simulink model "SixDOFSim"  (R2020b)
settings: Solver=VariableStepAuto  StartTime=0.0  StopTime=80  RelTol=1e-3
values from neighbouring files (symbols this model uses):
  A = sys_ol.A    [cost_condition_number.m]    (also in cost_coupling_control.m; cost_filter.m; coupling_control_scratch.m = sys.A; coupling_control_scratch2.m = sys.A)
  B = sys_ol.B    [cost_condition_number.m]    (also in cost_coupling_control.m; cost_filter.m; coupling_control_scratch.m = sys.B; coupling_control_scratch2.m = sys.B)
  C_tilde = zeros(size(C,1), size(A,1))    [SixDOFModel.m]    (also in cost_condition_number.m = struct_cond.C_tilde; cost_coupling_control.m = struct_cond.C_tilde; cost_filter.m = struct_cond.C_tilde; coupling_controller.m = T*C_resort)
  deltaX_init = Tx\deltaX_init    [SixDOFModel.m]    (also in coupling_controller_main.m = X_init-X_ap_simulink)
  eta_max = 15*pi/180    (= 0.261799387799)    [SixDOFModel.m]    (also in coupling_controller_main.m = 0.174532925199; load_messung_one_massmodel.m = 0.174532925199)
  eta_min = - 30*pi/180    (= -0.523598775598)    [SixDOFModel.m]    (also in coupling_controller_main.m = -0.436332312999; load_messung_one_massmodel.m = -0.436332312999)
  F = real(F)    [coupling_control_scratch.m]    (also in coupling_control_scratch2.m; coupling_controller.m = Kopt{end}; coupling_controller_main.m = -inv(C*(Ak\B)); coupling_controller_philipp.m = -inv(C*(Ak\B)))
  F_mod = F_ent(:,1:p/2)    [SixDOFModel.m]    (also in coupling_controller_main.m = F1*Q_mod; coupling_controller_philipp.m = F1*Q_mod; script_kein_theta_verk.m = F1*Q_mod)
  K_coupling = inv(Dstar)*compR    [SixDOFModel.m]    (also in coupling_controller_main.m = Kopt{1}; coupling_controller_philipp.m = Kopt{1}; script_kein_theta_verk.m = Kopt{1})
  latlon_init = [0;0]    [SixDOFModel.m]    (also in create_multi_model.m)
  m = i-1    [coupling_control_scratch.m]    (also in coupling_control_scratch2.m; defineABC.m = size(B_1,2) + size(B_2,2); implicit_linmod.m = length(U_ap); initializeParameters.m = 120000)
  noise_weight = [10 10 10 1 1 1 1 1 10 10 10 10 1 1 1 1 1 10]'    [SixDOFModel.m]
  P_e_init_1 = [0;0;-h_init_1]    [SixDOFModel.m]    (also in create_multi_model.m)
  P_e_init_2 = [0;0;-h_init_2]    [SixDOFModel.m]    (also in create_multi_model.m)
  q = X(5)    [nonlinear_6DOF.m]    (also in normieren.m = size (C,1))
  r = 5    [coupling_controller.m]    (also in coupling_controller_main.m = 100; coupling_controller_philipp.m = 200; nonlinear_6DOF.m = X(6); polgebiet.m = a2)
  sigmaf_max = 20*pi/180    (= 0.349065850399)    [SixDOFModel.m]    (also in coupling_controller_main.m; load_messung_one_massmodel.m)
  sigmaf_min = 0.5*pi/180    (= 0.00872664625997)    [SixDOFModel.m]    (also in coupling_controller_main.m; load_messung_one_massmodel.m)
  Tu = eye(size(B,2))    [SixDOFModel.m]    (also in normieren.m = zeros(p,p))
  Tx = eye(n)    [SixDOFModel.m]    (also in normieren.m = diag([200 15 50 0.1 0.1 0.1 45*pi/180 45*pi/180 10000 200 15)
  Ty = eye(size(C,1))    [SixDOFModel.m]    (also in normieren.m = zeros(q,q))
  U_ap = Tu\U_ap    [SixDOFModel.m]    (also in coupling_controller_main.m = AP(1,1).U_ap; create_multi_model.m = [U_ap_1;U_ap_2]; fsolve_trim.m = ap(11:14); trimValues.m = Z_ap(11:14))
  W_ap = W_ap(1:4)    [SixDOFModel.m]    (also in coupling_controller_philipp.m = (C*X_ap_simulink)')
  X_ap = [X_ap_1;X_ap_2]    [SixDOFModel.m]    (also in coupling_controller_main.m = AP(1,1).X_ap; create_multi_model.m; fsolve_trim.m = ap(1:10); trimValues.m = Z_ap(1:10))
  X_ap_simulink = Tx\X_ap_simulink    [SixDOFModel.m]    (also in coupling_controller_main.m = AP(1,1).X_ap_simulink; create_multi_model.m = [X_ap(1:8);X_ap(10);X_ap(11:18);X_ap(20)])
  X_init = Tx\X_init    [SixDOFModel.m]    (also in cost_coupling_control.m = struct_cond.X_init; cost_filter.m = struct_cond.X_init; coupling_controller_main.m = X_ap_simulink; create_multi_model.m = [X_init_1; X_init_2])
  xi_max = 25*pi/180    (= 0.436332312999)    [SixDOFModel.m]    (also in coupling_controller_main.m; load_messung_one_massmodel.m)
  xi_min = - xi_max    (= -0.436332312999)    [SixDOFModel.m]    (also in coupling_controller_main.m; load_messung_one_massmodel.m)
  zita_max = 30*pi/180    (= 0.523598775598)    [SixDOFModel.m]    (also in coupling_controller_main.m; load_messung_one_massmodel.m)
  zita_min = - zita_max    (= -0.523598775598)    [SixDOFModel.m]    (also in coupling_controller_main.m; load_messung_one_massmodel.m)
undefined symbols (not defined in the file or in its folder): Earth, globalParameters, Light, MIL, WGS84
libraries: aerolibfltsims x24, aerolibtransform2 x4, aerolibwind2 x4, simulink x3, shared6dof x1, aerolibanim x1
(part 2 of 3)

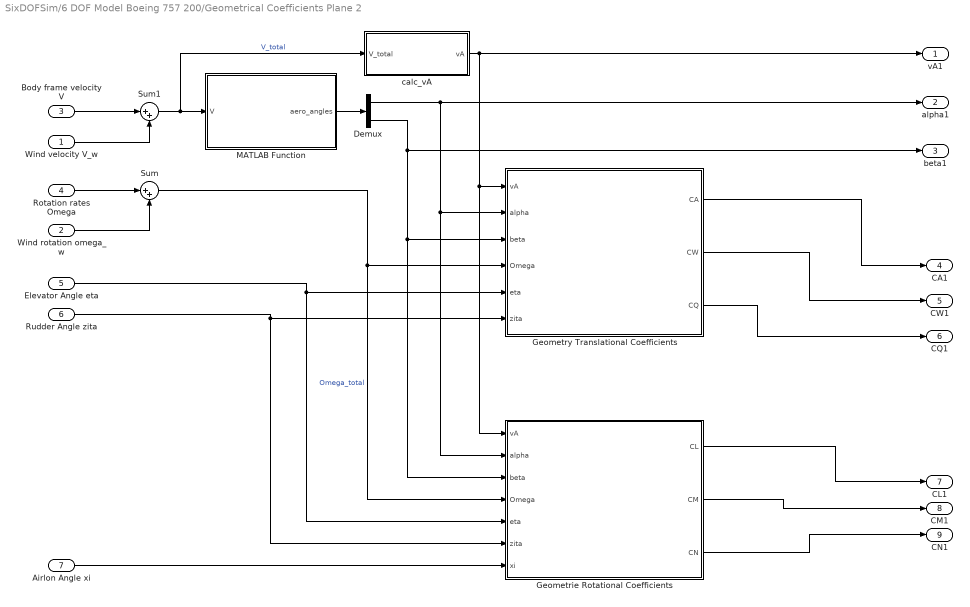
== system SixDOFSim/6 DOF Model Boeing 757 200/Geometrical Coefficients Plane 2 ==
  Wind velocity V_w : Inport
  Wind rotation omega_w : Inport  Port=2
  Body frame velocity V : Inport  Port=3
  Rotation rates Omega : Inport  Port=4
  Elevator Angle eta : Inport  Port=5
  Rudder Angle zita : Inport  Port=6
  Airlon Angle xi : Inport  Port=7
  Demux : Demux  Outputs=2
  Geometrie Rotational Coefficients : MATLAB Function  TreatAsAtomicUnit=on
  Geometry Translational Coefficients : MATLAB Function  TreatAsAtomicUnit=on
  MATLAB Function : MATLAB Function  TreatAsAtomicUnit=on
  Sum : Sum  Inputs=|++
  Sum1 : Sum  Inputs=|++
  calc_vA : MATLAB Function  TreatAsAtomicUnit=on
  vA1 : Outport
  alpha1 : Outport  Port=2
  beta1 : Outport  Port=3
  CA1 : Outport  Port=4
  CW1 : Outport  Port=5
  CQ1 : Outport  Port=6
  CL1 : Outport  Port=7
  CM1 : Outport  Port=8
  CN1 : Outport  Port=9
  wires:
  Airlon Angle xi/1 -> Geometrie Rotational Coefficients/7(xi)
  Geometrie Rotational Coefficients/2(CM) -> CM1/1
  Geometry Translational Coefficients/2(CW) -> CW1/1
  Rudder Angle zita/1 -> Geometrie Rotational Coefficients/6(zita), Geometry Translational Coefficients/6(zita)
  Geometry Translational Coefficients/1(CA) -> CA1/1
  Geometrie Rotational Coefficients/3(CN) -> CN1/1
  Geometry Translational Coefficients/3(CQ) -> CQ1/1
  Geometrie Rotational Coefficients/1(CL) -> CL1/1
  Elevator Angle eta/1 -> Geometrie Rotational Coefficients/5(eta), Geometry Translational Coefficients/5(eta)
  Body frame velocity V/1 -> Sum1/1
  Rotation rates Omega/1 -> Sum/1
  Wind velocity V_w/1 -> Sum1/2
  Wind rotation omega_w/1 -> Sum/2
  Sum1/1 -> calc_vA/1(V_total), MATLAB Function/1(V)  "V_total"
  MATLAB Function/1(aero_angles) -> Demux/1
  Demux/1 -> Geometrie Rotational Coefficients/2(alpha), Geometry Translational Coefficients/2(alpha), alpha1/1
  Demux/2 -> beta1/1, Geometrie Rotational Coefficients/3(beta), Geometry Translational Coefficients/3(beta)
  Sum/1 -> Geometrie Rotational Coefficients/4(Omega), Geometry Translational Coefficients/4(Omega)  "Omega_total"
  calc_vA/1(vA) -> vA1/1, Geometrie Rotational Coefficients/1(vA), Geometry Translational Coefficients/1(vA)

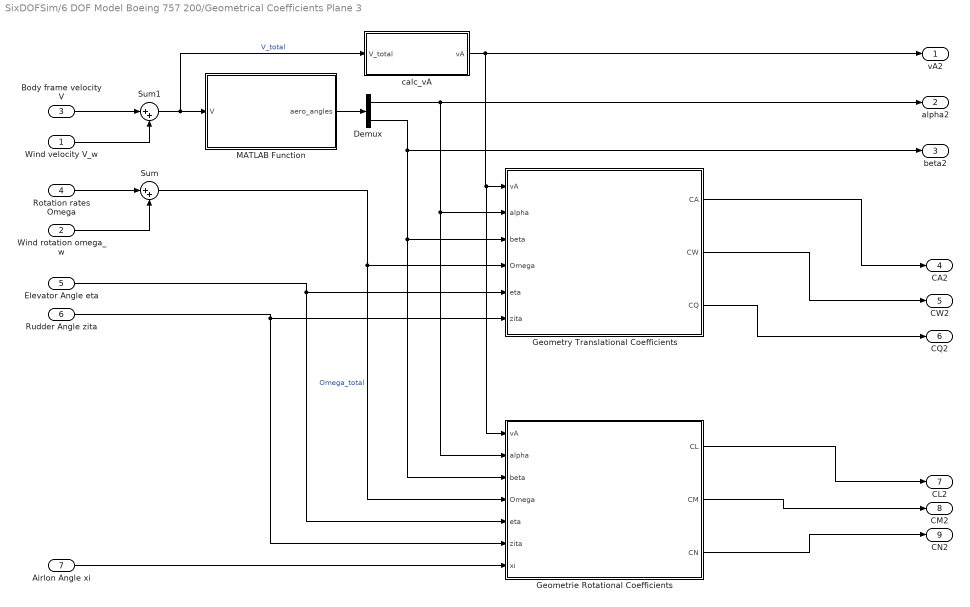
== system SixDOFSim/6 DOF Model Boeing 757 200/Geometrical Coefficients Plane 3 ==
  Wind velocity V_w : Inport
  Wind rotation omega_w : Inport  Port=2
  Body frame velocity V : Inport  Port=3
  Rotation rates Omega : Inport  Port=4
  Elevator Angle eta : Inport  Port=5
  Rudder Angle zita : Inport  Port=6
  Airlon Angle xi : Inport  Port=7
  Demux : Demux  Outputs=2
  Geometrie Rotational Coefficients : MATLAB Function  TreatAsAtomicUnit=on
  Geometry Translational Coefficients : MATLAB Function  TreatAsAtomicUnit=on
  MATLAB Function : MATLAB Function  TreatAsAtomicUnit=on
  Sum : Sum  Inputs=|++
  Sum1 : Sum  Inputs=|++
  calc_vA : MATLAB Function  TreatAsAtomicUnit=on
  vA2 : Outport
  alpha2 : Outport  Port=2
  beta2 : Outport  Port=3
  CA2 : Outport  Port=4
  CW2 : Outport  Port=5
  CQ2 : Outport  Port=6
  CL2 : Outport  Port=7
  CM2 : Outport  Port=8
  CN2 : Outport  Port=9
  wires:
  calc_vA/1(vA) -> Geometrie Rotational Coefficients/1(vA), Geometry Translational Coefficients/1(vA), vA2/1
  Sum/1 -> Geometry Translational Coefficients/4(Omega), Geometrie Rotational Coefficients/4(Omega)  "Omega_total"
  Demux/2 -> Geometry Translational Coefficients/3(beta), Geometrie Rotational Coefficients/3(beta), beta2/1
  Demux/1 -> alpha2/1, Geometry Translational Coefficients/2(alpha), Geometrie Rotational Coefficients/2(alpha)
  MATLAB Function/1(aero_angles) -> Demux/1
  Sum1/1 -> MATLAB Function/1(V), calc_vA/1(V_total)  "V_total"
  Wind rotation omega_w/1 -> Sum/2
  Wind velocity V_w/1 -> Sum1/2
  Rotation rates Omega/1 -> Sum/1
  Body frame velocity V/1 -> Sum1/1
  Elevator Angle eta/1 -> Geometry Translational Coefficients/5(eta), Geometrie Rotational Coefficients/5(eta)
  Geometrie Rotational Coefficients/1(CL) -> CL2/1
  Geometry Translational Coefficients/3(CQ) -> CQ2/1
  Geometrie Rotational Coefficients/3(CN) -> CN2/1
  Geometry Translational Coefficients/1(CA) -> CA2/1
  Rudder Angle zita/1 -> Geometry Translational Coefficients/6(zita), Geometrie Rotational Coefficients/6(zita)
  Geometry Translational Coefficients/2(CW) -> CW2/1
  Geometrie Rotational Coefficients/2(CM) -> CM2/1
  Airlon Angle xi/1 -> Geometrie Rotational Coefficients/7(xi)

== system SixDOFSim/6 DOF Model Boeing 757 200/Motion model Plain3 ==
  Omega : Inport
  V : Inport  Port=2
  Forces : Inport  Port=3
  Torque : Inport  Port=4
  Euler angles : Inport  Port=5
  Dynamics : Subsystem
  dV2 : Outport
  dOmega2 : Outport  Port=2
  dPhi2 : Outport  Port=3
  dxyh2 : Outport  Port=4
  vk2 : Outport  Port=5
  chsi2 : Outport  Port=6
  gamma2 : Outport  Port=7
  wires:
  Dynamics/7(gamma) -> gamma2/1
  Dynamics/6(chsi) -> chsi2/1
  Dynamics/5(vk) -> vk2/1
  Dynamics/4(dxyh) -> dxyh2/1
  Dynamics/3(dPhi) -> dPhi2/1
  Dynamics/1(dV) -> dV2/1
  V/1 -> Dynamics/2(V)
  Omega/1 -> Dynamics/1(Omega)
  Euler angles/1 -> Dynamics/5(Euler Angles( Phi))
  Torque/1 -> Dynamics/4(Torque)
  Forces/1 -> Dynamics/3(Forces)
  Dynamics/2(dOmega) -> dOmega2/1

== system SixDOFSim/6 DOF Model Boeing 757 200/Motion model Plane 2 ==
  Omega : Inport
  V : Inport  Port=2
  Forces : Inport  Port=3
  Torque : Inport  Port=4
  Euler angles : Inport  Port=5
  Dynamics : Subsystem
  dV1 : Outport
  dOmega1 : Outport  Port=2
  dPhi1 : Outport  Port=3
  dxyh1 : Outport  Port=4
  vk1 : Outport  Port=5
  chsi1 : Outport  Port=6
  gamma1 : Outport  Port=7
  wires:
  Dynamics/2(dOmega) -> dOmega1/1
  Forces/1 -> Dynamics/3(Forces)
  Torque/1 -> Dynamics/4(Torque)
  Euler angles/1 -> Dynamics/5(Euler Angles( Phi))
  Omega/1 -> Dynamics/1(Omega)
  V/1 -> Dynamics/2(V)
  Dynamics/1(dV) -> dV1/1
  Dynamics/3(dPhi) -> dPhi1/1
  Dynamics/4(dxyh) -> dxyh1/1
  Dynamics/5(vk) -> vk1/1
  Dynamics/6(chsi) -> chsi1/1
  Dynamics/7(gamma) -> gamma1/1

== system SixDOFSim/6 DOF Model Boeing 757 200/Rho ==
  h1 : Inport
  calc_rho : MATLAB Function  TreatAsAtomicUnit=on
  rho1 : Outport
  wires:
  h1/1 -> calc_rho/1(h)
  calc_rho/1(rho) -> rho1/1

== system SixDOFSim/6 DOF Model Boeing 757 200/Rho1 ==
  h2 : Inport
  calc_rho : MATLAB Function  TreatAsAtomicUnit=on
  rho2 : Outport
  wires:
  calc_rho/1(rho) -> rho2/1
  h2/1 -> calc_rho/1(h)

== system SixDOFSim/6 DOF Model Boeing 757 200/Stellgrößenbeschränkung ==
  eta_soll_1 : Inport
  sigmaf_soll_1 : Inport  Port=2
  xi_soll_1 : Inport  Port=3
  zita_soll_1 : Inport  Port=4
  Saturation airlon p1 : Saturate  UpperLimit=xi_max  LowerLimit=xi_min
  Saturation elevator p1 : Saturate  UpperLimit=eta_max  LowerLimit=eta_min
  Saturation rudder p1 : Saturate  UpperLimit=zita_max  LowerLimit=zita_min
  Saturation throttle p1 : Saturate  UpperLimit=sigmaf_max  LowerLimit=sigmaf_min
  eta_ist_1 : Outport
  sigmaf_ist_1 : Outport  Port=2
  xi_ist_1 : Outport  Port=3
  zita_ist_1 : Outport  Port=4
  wires:
  xi_soll_1/1 -> Saturation airlon p1/1
  zita_soll_1/1 -> Saturation rudder p1/1
  Saturation airlon p1/1 -> xi_ist_1/1
  Saturation elevator p1/1 -> eta_ist_1/1
  eta_soll_1/1 -> Saturation elevator p1/1
  Saturation throttle p1/1 -> sigmaf_ist_1/1
  sigmaf_soll_1/1 -> Saturation throttle p1/1
  Saturation rudder p1/1 -> zita_ist_1/1

== system SixDOFSim/6 DOF Model Boeing 757 200/Stellgrößenbeschränkung 2 ==
  eta_soll_2 : Inport
  sigmaf_soll_2 : Inport  Port=2
  xi_soll_2 : Inport  Port=3
  zita_soll_2 : Inport  Port=4
  Saturation airlon p2 : Saturate  UpperLimit=xi_max  LowerLimit=xi_min
  Saturation elevator p2 : Saturate  UpperLimit=eta_max  LowerLimit=eta_min
  Saturation rudder p2 : Saturate  UpperLimit=zita_max  LowerLimit=zita_min
  Saturation throttle p2 : Saturate  UpperLimit=sigmaf_max  LowerLimit=sigmaf_min
  eta_ist_2 : Outport
  sigmaf_ist_2 : Outport  Port=2
  xi_ist_2 : Outport  Port=3
  zita_ist_2 : Outport  Port=4
  wires:
  Saturation throttle p2/1 -> sigmaf_ist_2/1
  Saturation elevator p2/1 -> eta_ist_2/1
  sigmaf_soll_2/1 -> Saturation throttle p2/1
  Saturation airlon p2/1 -> xi_ist_2/1
  eta_soll_2/1 -> Saturation elevator p2/1
  xi_soll_2/1 -> Saturation airlon p2/1
  Saturation rudder p2/1 -> zita_ist_2/1
  zita_soll_2/1 -> Saturation rudder p2/1

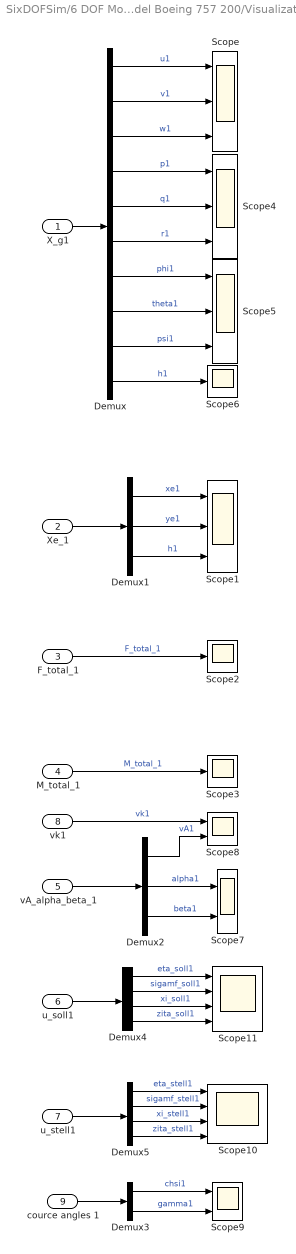
== system SixDOFSim/6 DOF Model Boeing 757 200/Visualization ==
  X_g1 : Inport
  Xe_1 : Inport  Port=2
  F_total_1 : Inport  Port=3
  M_total_1 : Inport  Port=4
  vA_alpha_beta_1 : Inport  Port=5
  u_soll1 : Inport  Port=6
  u_stell1 : Inport  Port=7
  vk1 : Inport  Port=8
  cource angles 1 : Inport  Port=9
  Demux : Demux  Outputs=10
  Demux1 : Demux  Outputs=3
  Demux2 : Demux  Outputs=3
  Demux3 : Demux  Outputs=2
  Demux4 : Demux
  Demux5 : Demux
  Scope{,1,4..5} (4 alike) : Scope  NumInputPorts=3
  Scope10 : Scope  NumInputPorts=4
  Scope11 : Scope  NumInputPorts=4
  Scope2 : Scope
  Scope3 : Scope
  Scope6 : Scope
  Scope7 : Scope  NumInputPorts=2
  Scope8 : Scope  NumInputPorts=2
  Scope9 : Scope  NumInputPorts=2
  wires:
  Xe_1/1 -> Demux1/1
  X_g1/1 -> Demux/1
  F_total_1/1 -> Scope2/1  "F_total_1"
  M_total_1/1 -> Scope3/1  "M_total_1"
  Demux/1 -> Scope/1  "u1"
  Demux/2 -> Scope/2  "v1"
  Demux/3 -> Scope/3  "w1"
  Demux/5 -> Scope4/2  "q1"
  Demux/4 -> Scope4/1  "p1"
  Demux/6 -> Scope4/3  "r1"
  Demux/7 -> Scope5/1  "phi1"
  Demux/8 -> Scope5/2  "theta1"
  Demux/9 -> Scope5/3  "psi1"
  Demux/10 -> Scope6/1  "h1"
  Demux1/2 -> Scope1/2  "ye1"
  Demux1/1 -> Scope1/1  "xe1"
  Demux1/3 -> Scope1/3  "h1"
  Demux2/3 -> Scope7/2  "beta1"
  Demux2/2 -> Scope7/1  "alpha1"
  vA_alpha_beta_1/1 -> Demux2/1
  vk1/1 -> Scope8/1  "vk1"
  Demux2/1 -> Scope8/2  "vA1"
  cource angles 1/1 -> Demux3/1
  Demux3/1 -> Scope9/1  "chsi1"
  Demux3/2 -> Scope9/2  "gamma1"
  u_stell1/1 -> Demux5/1
  Demux5/1 -> Scope10/1  "eta_stell1"
  Demux5/2 -> Scope10/2  "sigamf_stell1"
  Demux5/3 -> Scope10/3  "xi_stell1"
  u_soll1/1 -> Demux4/1
  Demux4/1 -> Scope11/1  "eta_soll1"
  Demux4/2 -> Scope11/2  "sigamf_soll1"
  Demux4/3 -> Scope11/3  "xi_soll1"
  Demux4/4 -> Scope11/4  "zita_soll1"
  Demux5/4 -> Scope10/4  "zita_stell1"

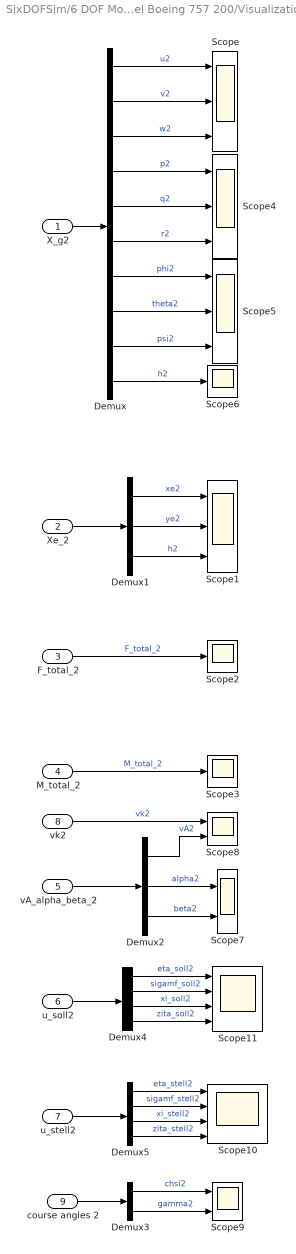
== system SixDOFSim/6 DOF Model Boeing 757 200/Visualization1 ==
  X_g2 : Inport
  Xe_2 : Inport  Port=2
  F_total_2 : Inport  Port=3
  M_total_2 : Inport  Port=4
  vA_alpha_beta_2 : Inport  Port=5
  u_soll2 : Inport  Port=6
  u_stell2 : Inport  Port=7
  vk2 : Inport  Port=8
  course angles 2 : Inport  Port=9
  Demux : Demux  Outputs=10
  Demux1 : Demux  Outputs=3
  Demux2 : Demux  Outputs=3
  Demux3 : Demux  Outputs=2
  Demux4 : Demux
  Demux5 : Demux
  Scope{,1,4..5} (4 alike) : Scope  NumInputPorts=3
  Scope10 : Scope  NumInputPorts=4
  Scope11 : Scope  NumInputPorts=4
  Scope2 : Scope
  Scope3 : Scope
  Scope6 : Scope
  Scope7 : Scope  NumInputPorts=2
  Scope8 : Scope  NumInputPorts=2
  Scope9 : Scope  NumInputPorts=2
  wires:
  Demux5/4 -> Scope10/4  "zita_stell2"
  Demux4/4 -> Scope11/4  "zita_soll2"
  Demux4/3 -> Scope11/3  "xi_soll2"
  Demux4/2 -> Scope11/2  "sigamf_soll2"
  Demux4/1 -> Scope11/1  "eta_soll2"
  u_soll2/1 -> Demux4/1
  Demux5/3 -> Scope10/3  "xi_stell2"
  Demux5/2 -> Scope10/2  "sigamf_stell2"
  Demux5/1 -> Scope10/1  "eta_stell2"
  u_stell2/1 -> Demux5/1
  Demux3/2 -> Scope9/2  "gamma2"
  Demux3/1 -> Scope9/1  "chsi2"
  course angles 2/1 -> Demux3/1
  Demux2/1 -> Scope8/2  "vA2"
  vk2/1 -> Scope8/1  "vk2"
  vA_alpha_beta_2/1 -> Demux2/1
  Demux2/2 -> Scope7/1  "alpha2"
  Demux2/3 -> Scope7/2  "beta2"
  Demux1/3 -> Scope1/3  "h2"
  Demux1/1 -> Scope1/1  "xe2"
  Demux1/2 -> Scope1/2  "ye2"
  Demux/10 -> Scope6/1  "h2"
  Demux/9 -> Scope5/3  "psi2"
  Demux/8 -> Scope5/2  "theta2"
  Demux/7 -> Scope5/1  "phi2"
  Demux/6 -> Scope4/3  "r2"
  Demux/4 -> Scope4/1  "p2"
  Demux/5 -> Scope4/2  "q2"
  Demux/3 -> Scope/3  "w2"
  Demux/2 -> Scope/2  "v2"
  Demux/1 -> Scope/1  "u2"
  M_total_2/1 -> Scope3/1  "M_total_2"
  F_total_2/1 -> Scope2/1  "F_total_2"
  X_g2/1 -> Demux/1
  Xe_2/1 -> Demux1/1

== system SixDOFSim/6 DOF Model Boeing 757 200/Wind ==
  Airspeed : Inport
  Altitude : Inport  Port=2
  DCM : Inport  Port=3
  Discrete Wind Gust Model : aerolibwind2/Discrete Wind Gust Model  units=Metric (MKS)  Gx=on  Gy=on  Gz=on  t_0=5  d_m=[120 120 80]  v_m=[3.5 3.5 3.0]
  Dryden Wind Turbulence Model (Discrete (+q +r)) : aerolibwind2/Dryden Wind Turbulence Model  (Continuous (+q -r))  units=Metric (MKS)  spec=MIL-F-8785C  model=Discrete Dryden (+q +r)  W20=15  Wdeg=0  TurbProb=10^-2 - Light  L_high=533.4  Wingspan=10  ts=0.1  Seed=[23341 23342 23343 23344]  T_on=on
  Sum : Sum  Inputs=|++
  abs(V) : MATLAB Function  TreatAsAtomicUnit=on
  V_w1 : Outport
  pg1,qg1,rg1 : Outport  Port=2
  wires:
  Altitude/1 -> Dryden Wind Turbulence Model (Discrete (+q +r))/1
  Discrete Wind Gust Model/1 -> Sum/1
  Sum/1 -> V_w1/1
  Dryden Wind Turbulence Model (Discrete (+q +r))/1 -> Sum/2
  Dryden Wind Turbulence Model (Discrete (+q +r))/2 -> pg1,qg1,rg1/1
  DCM/1 -> Dryden Wind Turbulence Model (Discrete (+q +r))/3
  Airspeed/1 -> abs(V)/1(u)
  abs(V)/1(y) -> Dryden Wind Turbulence Model (Discrete (+q +r))/2, Discrete Wind Gust Model/1

== system SixDOFSim/6 DOF Model Boeing 757 200/Wind1 ==
  Airspeed : Inport
  Altitude : Inport  Port=2
  DCM : Inport  Port=3
  Discrete Wind Gust Model : aerolibwind2/Discrete Wind Gust Model  units=Metric (MKS)  Gx=on  Gy=on  Gz=on  t_0=5  d_m=[120 120 80]  v_m=[3.5 3.5 3.0]
  Dryden Wind Turbulence Model (Discrete (+q +r)) : aerolibwind2/Dryden Wind Turbulence Model  (Continuous (+q -r))  units=Metric (MKS)  spec=MIL-F-8785C  model=Discrete Dryden (+q +r)  W20=15  Wdeg=0  TurbProb=10^-2 - Light  L_high=533.4  Wingspan=10  ts=0.1  Seed=[23341 23342 23343 23344]  T_on=on
  Sum : Sum  Inputs=|++
  abs(V) : MATLAB Function  TreatAsAtomicUnit=on
  V_w2 : Outport
  pg2,qg2,rg2 : Outport  Port=2
  wires:
  DCM/1 -> Dryden Wind Turbulence Model (Discrete (+q +r))/3
  Dryden Wind Turbulence Model (Discrete (+q +r))/2 -> pg2,qg2,rg2/1
  Dryden Wind Turbulence Model (Discrete (+q +r))/1 -> Sum/2
  Sum/1 -> V_w2/1
  Discrete Wind Gust Model/1 -> Sum/1
  Altitude/1 -> Dryden Wind Turbulence Model (Discrete (+q +r))/1
  Airspeed/1 -> abs(V)/1(u)
  abs(V)/1(y) -> Dryden Wind Turbulence Model (Discrete (+q +r))/2, Discrete Wind Gust Model/1

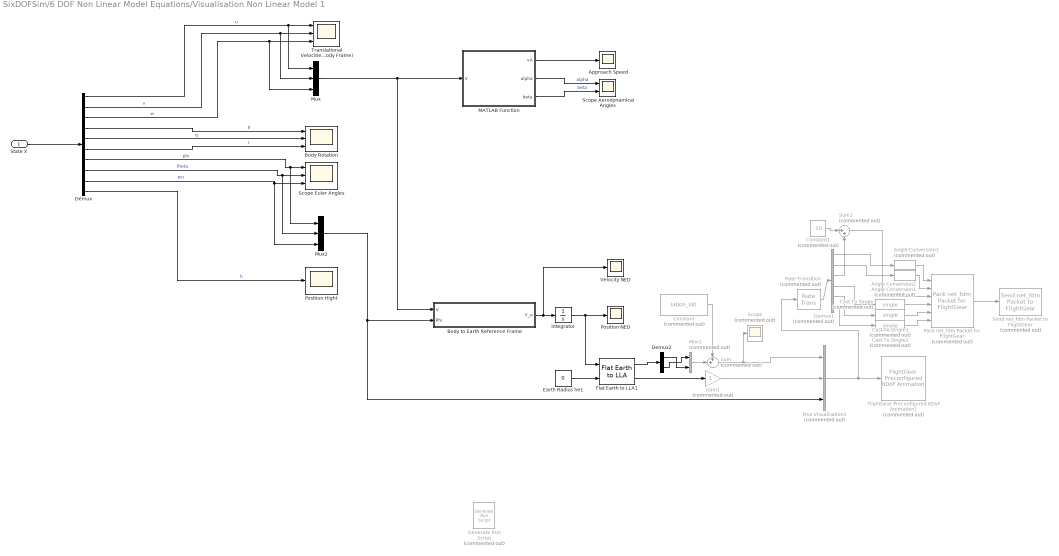
== system SixDOFSim/6 DOF Non Linear Model Equations/Visualisation Non Linear Model 1 ==
  State X : Inport
  Angle Conversion1 : aerolibfltsims/FlightGear Preconfigured 6DoF Animation/Angle Conversion1  Commented=on  SystemSampleTime=-1  VariantActivationTime=update diagram  Latency=0  AutoFrameSizeCalculation=off
      settings: SourceProductBaseCode=AE
  Angle Conversion2 : aerolibfltsims/FlightGear Preconfigured 6DoF Animation/Angle Conversion1  Commented=on  SystemSampleTime=-1  VariantActivationTime=update diagram  Latency=0  AutoFrameSizeCalculation=off
      settings: SourceProductBaseCode=AE
  Approach Speed : Scope
  Body Rotation : Scope  NumInputPorts=3
  "Body to Earth Reference Frame " : MATLAB Function  TreatAsAtomicUnit=on
  Cast To Single : DataTypeConversion  Commented=on  OutDataTypeStr=single
  Cast To Single1 : DataTypeConversion  Commented=on  OutDataTypeStr=single
  Cast To Single2 : DataTypeConversion  Commented=on  OutDataTypeStr=single
  Constant : Constant  Commented=on  Value=latlon_init
  Constant1 : Constant  Commented=on  Value=-10
  Demux : Demux  Outputs=10
  Demux1 : Demux  Commented=on  Outputs=6
  Demux2 : Demux  Outputs=2
  Earth Radius he1 : Constant  Value=0
  Flat Earth to LLA1 : aerolibtransform2/Flat Earth to LLA  units=Metric (MKS)  ptype=Earth (WGS84)  F=1/298.257223563  R=6378137  refPosPort=off  LL0=[0 10]  psi=0
  FlightGear Preconfigured 6DoF Animation1 : aerolibfltsims/FlightGear Preconfigured 6DoF Animation  Commented=on  xFlightGearVersion=v2019.1  DestinationIpAddress=127.0.0.1  DestinationPort=5502  SampleTime=1/30  packetVersion=24
  Gain1 : Gain  Commented=on
  Generate Run Script : aerolibfltsims/Generate Run Script  Commented=on  Architecture=Win64  dataFlow=Send  GeometryModelName=c172p  AirportId=KSFO  RunwayId=10L  InitialAltitude=7224  InitialHeading=113  OffsetDistance=4.72  OffsetAzimuth=0  InstallScenery=off  DisableShaders=on  OriginAddress=127.0.0.1  DestinationPort=5502  OriginPort=5505  LocalAddress=127.0.0.1  OutputFileName=runfg.bat  FlightGearBaseDirectory=D:\Flight Gear\FlightGear 2018.1.1
  Integrator : Integrator  InitialCondition=P_e_init_1
  MATLAB Function : MATLAB Function  TreatAsAtomicUnit=on
  Mux : Mux  Inputs=3
  Mux Visualisation1 : Mux  Commented=on  Inputs=3
  Mux1 : Mux  Commented=on  Inputs=2
  Mux2 : Mux  Inputs=3
  Pack net_fdm Packet for FlightGear : aerolibfltsims/Pack net_fdm Packet for FlightGear  Commented=on  FlightGearVersion=v2019.1  ShowPositionAttitudeInputs=on  ShowVelocityAccelerationInputs=off  ShowControlSurfacePositionInputs=off  ShowEngineFuelInputs=off  ShowLandingGearInputs=off  ShowEnvironmentInputs=off  SampleTime=1/30  packetVersion=24
      settings: SourceProductBaseCode=AE
  Position Hight : Scope
  Position NED : Scope
  Rate Transition : RateTransition  Commented=on  Integrity=off  Deterministic=off
  Scope : Scope  Commented=on
  Scope Aerodynamical Angles : Scope  NumInputPorts=2
  Scope Euler Angles : Scope  NumInputPorts=3
  Send net_fdm Packet to FlightGear : aerolibfltsims/Send net_fdm Packet to FlightGear  Commented=on  DestinationIpAddress=127.0.0.1  DestinationPort=5503  LocalIpPort=-1  varLen=off  SampleTime=1/30
      settings: SourceProductBaseCode=AE
  Sum : Sum  Commented=on  Inputs=++|
  Sum1 : Sum  Commented=on  Inputs=|++
  Translational Velocities (Body Frame) : Scope  NumInputPorts=3
  Velocity NED : Scope
  wires:
  State X/1 -> Demux/1
  Demux2/2 -> Mux1/1
  Flat Earth to LLA1/2 -> Gain1/1
  Gain1/1 -> Mux Visualisation1/2
  Mux Visualisation1/1 -> FlightGear Preconfigured 6DoF Animation1/1, Rate Transition/1
  Earth Radius he1/1 -> Flat Earth to LLA1/2
  Flat Earth to LLA1/1 -> Demux2/1
  Demux2/1 -> Mux1/2
  "Body to Earth Reference Frame "/1(V_e) -> Velocity NED/1, Integrator/1
  Integrator/1 -> Position NED/1, Flat Earth to LLA1/1
  Demux/1 -> Mux/1, Translational Velocities (Body Frame)/1  "u"
  Demux/2 -> Mux/2, Translational Velocities (Body Frame)/2  "v"
  Demux/3 -> Translational Velocities (Body Frame)/3, Mux/3  "w"
  Demux/4 -> Body Rotation/1  "p"
  Demux/5 -> Body Rotation/2  "q"
  Demux/6 -> Body Rotation/3  "r"
  Demux/7 -> Mux2/1, Scope Euler Angles/1  "phi"
  Demux/8 -> Mux2/2, Scope Euler Angles/2  "theta"
  Demux/9 -> Mux2/3, Scope Euler Angles/3  "psi"
  Demux/10 -> Position Hight/1  "h"
  Mux/1 -> MATLAB Function/1(V), "Body to Earth Reference Frame "/1(V)
  Mux2/1 -> "Body to Earth Reference Frame "/2(Phi), Mux Visualisation1/3
  MATLAB Function/1(vA) -> Approach Speed/1
  MATLAB Function/2(alpha) -> Scope Aerodynamical Angles/1  "alpha"
  MATLAB Function/3(beta) -> Scope Aerodynamical Angles/2  "beta"
  Mux1/1 -> Sum/2
  Sum/1 -> Scope/1, Mux Visualisation1/1
  Constant/1 -> Sum/1
  Pack net_fdm Packet for FlightGear/1 -> Send net_fdm Packet to FlightGear/1
  Angle Conversion1/1 -> Pack net_fdm Packet for FlightGear/1
  Angle Conversion2/1 -> Pack net_fdm Packet for FlightGear/2
  Cast To Single/1 -> Pack net_fdm Packet for FlightGear/4
  Cast To Single1/1 -> Pack net_fdm Packet for FlightGear/5
  Cast To Single2/1 -> Pack net_fdm Packet for FlightGear/6
  Demux1/2 -> Angle Conversion2/1
  Rate Transition/1 -> Demux1/1
  Demux1/1 -> Angle Conversion1/1
  Constant1/1 -> Sum1/1
  Demux1/3 -> Sum1/2
  Sum1/1 -> Pack net_fdm Packet for FlightGear/3
  Demux1/4 -> Cast To Single/1
  Demux1/5 -> Cast To Single1/1
  Demux1/6 -> Cast To Single2/1

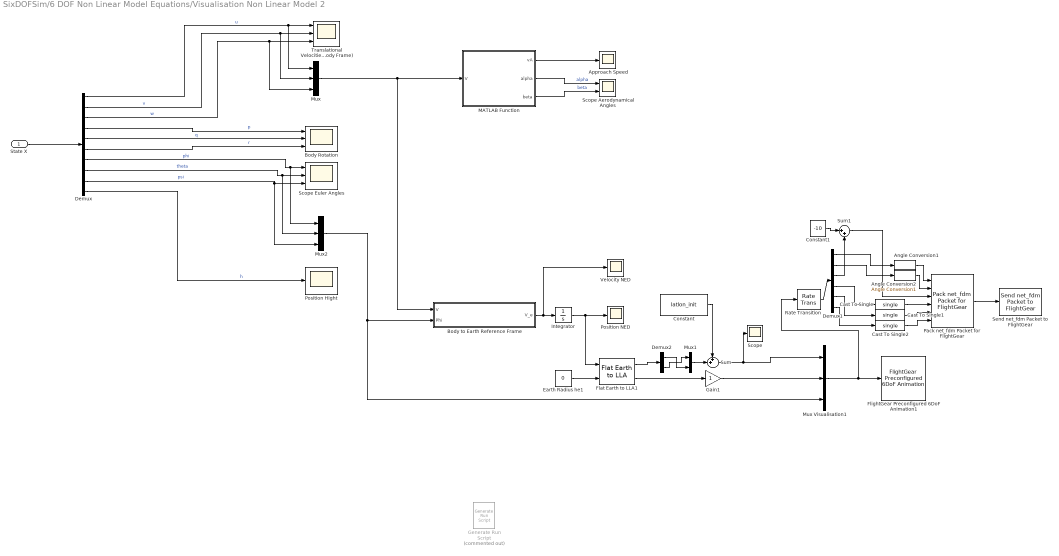
== system SixDOFSim/6 DOF Non Linear Model Equations/Visualisation Non Linear Model 2 ==
  State X : Inport
  Angle Conversion1 : aerolibfltsims/FlightGear Preconfigured 6DoF Animation/Angle Conversion1  SystemSampleTime=-1  VariantActivationTime=update diagram  Latency=0  AutoFrameSizeCalculation=off
      settings: SourceProductBaseCode=AE
  Angle Conversion2 : aerolibfltsims/FlightGear Preconfigured 6DoF Animation/Angle Conversion1  SystemSampleTime=-1  VariantActivationTime=update diagram  Latency=0  AutoFrameSizeCalculation=off
      settings: SourceProductBaseCode=AE
  Approach Speed : Scope
  Body Rotation : Scope  NumInputPorts=3
  "Body to Earth Reference Frame " : MATLAB Function  TreatAsAtomicUnit=on
  Cast To Single : DataTypeConversion  OutDataTypeStr=single
  Cast To Single1 : DataTypeConversion  OutDataTypeStr=single
  Cast To Single2 : DataTypeConversion  OutDataTypeStr=single
  Constant : Constant  Value=latlon_init
  Constant1 : Constant  Value=-10
  Demux : Demux  Outputs=10
  Demux1 : Demux  Outputs=6
  Demux2 : Demux  Outputs=2
  Earth Radius he1 : Constant  Value=0
  Flat Earth to LLA1 : aerolibtransform2/Flat Earth to LLA  units=Metric (MKS)  ptype=Earth (WGS84)  F=1/298.257223563  R=6378137  refPosPort=off  LL0=[0 10]  psi=0
  FlightGear Preconfigured 6DoF Animation1 : aerolibfltsims/FlightGear Preconfigured 6DoF Animation  xFlightGearVersion=v2019.1  DestinationIpAddress=127.0.0.1  DestinationPort=5502  SampleTime=1/30  packetVersion=24
  Gain1 : Gain
  Generate Run Script : aerolibfltsims/Generate Run Script  Commented=on  Architecture=Win64  dataFlow=Send  GeometryModelName=c172p  AirportId=KSFO  RunwayId=10L  InitialAltitude=7224  InitialHeading=113  OffsetDistance=4.72  OffsetAzimuth=0  InstallScenery=off  DisableShaders=on  OriginAddress=127.0.0.1  DestinationPort=5502  OriginPort=5505  LocalAddress=127.0.0.1  OutputFileName=runfg.bat  FlightGearBaseDirectory=D:\Flight Gear\FlightGear 2018.1.1
  Integrator : Integrator  InitialCondition=P_e_init_2
  MATLAB Function : MATLAB Function  TreatAsAtomicUnit=on
  Mux : Mux  Inputs=3
  Mux Visualisation1 : Mux  Inputs=3
  Mux1 : Mux  Inputs=2
  Mux2 : Mux  Inputs=3
  Pack net_fdm Packet for FlightGear : aerolibfltsims/Pack net_fdm Packet for FlightGear  FlightGearVersion=v2019.1  ShowPositionAttitudeInputs=on  ShowVelocityAccelerationInputs=off  ShowControlSurfacePositionInputs=off  ShowEngineFuelInputs=off  ShowLandingGearInputs=off  ShowEnvironmentInputs=off  SampleTime=1/30  packetVersion=24
      settings: SourceProductBaseCode=AE
  Position Hight : Scope
  Position NED : Scope
  Rate Transition : RateTransition  Integrity=off  Deterministic=off
  Scope : Scope
  Scope Aerodynamical Angles : Scope  NumInputPorts=2
  Scope Euler Angles : Scope  NumInputPorts=3
  Send net_fdm Packet to FlightGear : aerolibfltsims/Send net_fdm Packet to FlightGear  DestinationIpAddress=127.0.0.1  DestinationPort=5503  LocalIpPort=-1  varLen=off  SampleTime=1/30
      settings: SourceProductBaseCode=AE
  Sum : Sum  Inputs=++|
  Sum1 : Sum  Inputs=|++
  Translational Velocities (Body Frame) : Scope  NumInputPorts=3
  Velocity NED : Scope
  wires:
  State X/1 -> Demux/1
  Demux2/2 -> Mux1/1
  Flat Earth to LLA1/2 -> Gain1/1
  Gain1/1 -> Mux Visualisation1/2
  Mux Visualisation1/1 -> FlightGear Preconfigured 6DoF Animation1/1, Rate Transition/1
  Earth Radius he1/1 -> Flat Earth to LLA1/2
  Flat Earth to LLA1/1 -> Demux2/1
  Demux2/1 -> Mux1/2
  "Body to Earth Reference Frame "/1(V_e) -> Velocity NED/1, Integrator/1
  Integrator/1 -> Position NED/1, Flat Earth to LLA1/1
  Demux/1 -> Mux/1, Translational Velocities (Body Frame)/1  "u"
  Demux/2 -> Mux/2, Translational Velocities (Body Frame)/2  "v"
  Demux/3 -> Translational Velocities (Body Frame)/3, Mux/3  "w"
  Demux/4 -> Body Rotation/1  "p"
  Demux/5 -> Body Rotation/2  "q"
  Demux/6 -> Body Rotation/3  "r"
  Demux/7 -> Mux2/1, Scope Euler Angles/1  "phi"
  Demux/8 -> Mux2/2, Scope Euler Angles/2  "theta"
  Demux/9 -> Mux2/3, Scope Euler Angles/3  "psi"
  Demux/10 -> Position Hight/1  "h"
  Mux/1 -> MATLAB Function/1(V), "Body to Earth Reference Frame "/1(V)
  Mux2/1 -> "Body to Earth Reference Frame "/2(Phi), Mux Visualisation1/3
  MATLAB Function/1(vA) -> Approach Speed/1
  MATLAB Function/2(alpha) -> Scope Aerodynamical Angles/1  "alpha"
  MATLAB Function/3(beta) -> Scope Aerodynamical Angles/2  "beta"
  Mux1/1 -> Sum/2
  Sum/1 -> Scope/1, Mux Visualisation1/1
  Constant/1 -> Sum/1
  Pack net_fdm Packet for FlightGear/1 -> Send net_fdm Packet to FlightGear/1
  Angle Conversion1/1 -> Pack net_fdm Packet for FlightGear/1
  Angle Conversion2/1 -> Pack net_fdm Packet for FlightGear/2
  Cast To Single/1 -> Pack net_fdm Packet for FlightGear/4
  Cast To Single1/1 -> Pack net_fdm Packet for FlightGear/5
  Cast To Single2/1 -> Pack net_fdm Packet for FlightGear/6
  Demux1/2 -> Angle Conversion2/1
  Rate Transition/1 -> Demux1/1
  Demux1/1 -> Angle Conversion1/1
  Constant1/1 -> Sum1/1
  Demux1/3 -> Sum1/2
  Sum1/1 -> Pack net_fdm Packet for FlightGear/3
  Demux1/4 -> Cast To Single/1
  Demux1/5 -> Cast To Single1/1
  Demux1/6 -> Cast To Single2/1

== system SixDOFSim/6 DOF Model Boeing 757 200/Motion model Plain3/Dynamics ==
  Omega : Inport
  V : Inport  Port=2
  Forces : Inport  Port=3
  Torque : Inport  Port=4
  Euler Angles( Phi) : Inport  Port=5
  Divide : Product  Commented=on  Inputs=*/
  MATLAB Function : MATLAB Function  TreatAsAtomicUnit=on
  Sum : Sum  Commented=on  Inputs=+|+
  Terminator : Terminator
  Total mass of plane 1 (Betanker) : Subsystem  Commented=on
  Track and Aerodynamical Speed : MATLAB Function  TreatAsAtomicUnit=on
  Transformation of gravity in (Körperfestes System) : MATLAB Function  Commented=on  TreatAsAtomicUnit=on
  dV : Outport
  dOmega : Outport  Port=2
  dPhi : Outport  Port=3
  dxyh : Outport  Port=4
  vk : Outport  Port=5
  chsi : Outport  Port=6
  gamma : Outport  Port=7
  wires:
  Track and Aerodynamical Speed/1(dxyh) -> dxyh/1
  Track and Aerodynamical Speed/2(vk) -> vk/1
  Track and Aerodynamical Speed/4(chsi) -> chsi/1
  Track and Aerodynamical Speed/3(gamma) -> gamma/1
  MATLAB Function/1(dV) -> dV/1
  MATLAB Function/3(dPhi) -> dPhi/1
  V/1 -> Track and Aerodynamical Speed/2(V), MATLAB Function/3(V)
  Omega/1 -> MATLAB Function/2(Omega)
  Euler Angles( Phi)/1 -> MATLAB Function/1(Phi), Track and Aerodynamical Speed/1(Phi)
  Transformation of gravity in (Körperfestes System)/1(gravityAcceleration) -> Sum/1
  Forces/1 -> MATLAB Function/4(R_total)
  Sum/1 -> Terminator/1
  Divide/1 -> Sum/2
  Torque/1 -> MATLAB Function/5(Q_total)
  MATLAB Function/2(dOmega) -> dOmega/1
  Total mass of plane 1 (Betanker)/1(m_total) -> Divide/2

== system SixDOFSim/6 DOF Model Boeing 757 200/Motion model Plane 2/Dynamics ==
  Omega : Inport
  V : Inport  Port=2
  Forces : Inport  Port=3
  Torque : Inport  Port=4
  Euler Angles( Phi) : Inport  Port=5
  Divide : Product  Commented=on  Inputs=*/
  MATLAB Function : MATLAB Function  TreatAsAtomicUnit=on
  Sum : Sum  Commented=on  Inputs=+|+
  Total mass of plane 1 (Betanker) : Subsystem  Commented=on
  Track and Aerodynamical Speed : MATLAB Function  TreatAsAtomicUnit=on
  Transformation of gravity in (Körperfestes System) : MATLAB Function  Commented=on  TreatAsAtomicUnit=on
  dV : Outport
  dOmega : Outport  Port=2
  dPhi : Outport  Port=3
  dxyh : Outport  Port=4
  vk : Outport  Port=5
  chsi : Outport  Port=6
  gamma : Outport  Port=7
  wires:
  Total mass of plane 1 (Betanker)/1(m_total) -> Divide/2
  MATLAB Function/2(dOmega) -> dOmega/1
  Torque/1 -> MATLAB Function/5(Q_total)
  Divide/1 -> Sum/2
  Forces/1 -> MATLAB Function/4(R_total)
  Transformation of gravity in (Körperfestes System)/1(gravityAcceleration) -> Sum/1
  Euler Angles( Phi)/1 -> Track and Aerodynamical Speed/1(Phi), MATLAB Function/1(Phi)
  Omega/1 -> MATLAB Function/2(Omega)
  V/1 -> Track and Aerodynamical Speed/2(V), MATLAB Function/3(V)
  MATLAB Function/3(dPhi) -> dPhi/1
  MATLAB Function/1(dV) -> dV/1
  Track and Aerodynamical Speed/3(gamma) -> gamma/1
  Track and Aerodynamical Speed/4(chsi) -> chsi/1
  Track and Aerodynamical Speed/2(vk) -> vk/1
  Track and Aerodynamical Speed/1(dxyh) -> dxyh/1

== system SixDOFSim/6 DOF Model Boeing 757 200/Motion model Plain3/Dynamics/Total mass of plane 1 (Betanker) ==
  Constant : Constant  Value=m+globalParameters.m_fuel
  Constant1 : Constant  Value=0
  Constant2 : Constant  Value=globalParameters.refuel
  Ramp : simulink/Sources/Ramp  slope=globalParameters.m_fuel/globalParameters.time_refuel  start=globalParameters.start_time_refuel  InitialOutput=0  VectorParams1D=off
  Saturation : Saturate  UpperLimit=globalParameters.m_fuel  LowerLimit=0
  Scope : Scope
  Sum2 : Sum  Inputs=|+-
  Switch : Switch  Criteria=u2 > Threshold
  m_total : Outport
  wires:
  Switch/1 -> Sum2/2
  Constant2/1 -> Switch/2
  Ramp/1 -> Saturation/1
  Saturation/1 -> Switch/3
  Constant1/1 -> Switch/1
  Constant/1 -> Sum2/1
  Sum2/1 -> Scope/1, m_total/1

== system SixDOFSim/6 DOF Model Boeing 757 200/Motion model Plane 2/Dynamics/Total mass of plane 1 (Betanker) ==
  Constant : Constant  Value=m+globalParameters.m_fuel
  Constant1 : Constant  Value=0
  Constant2 : Constant  Value=globalParameters.refuel
  Ramp : simulink/Sources/Ramp  slope=globalParameters.m_fuel/globalParameters.time_refuel  start=globalParameters.start_time_refuel  InitialOutput=0  VectorParams1D=off
  Saturation : Saturate  UpperLimit=globalParameters.m_fuel  LowerLimit=0
  Scope : Scope
  Sum2 : Sum  Inputs=|+-
  Switch : Switch  Criteria=u2 > Threshold
  m_total : Outport
  wires:
  Sum2/1 -> m_total/1, Scope/1
  Constant/1 -> Sum2/1
  Constant1/1 -> Switch/1
  Saturation/1 -> Switch/3
  Ramp/1 -> Saturation/1
  Constant2/1 -> Switch/2
  Switch/1 -> Sum2/2

== matlab function SixDOFSim/6 DOF Non Linear Model Equations/Visualisation Non Linear Model 2/MATLAB Function ==
  data: V input; vA output; alpha output; beta output
function [vA,alpha,beta] = getAerodynamical(V)
u = V(1);
v = V(2);
w = V(3);
vA = sqrt(u^2+v^2+w^2);
alpha = atan2(w,u);
beta = asin(v/vA);

== matlab function SixDOFSim/6 DOF Linear/Visualisation Non Linear Model Plain 1/Body to Earth Reference Frame  ==
  data: V input; Phi input; V_e output
function V_e = getEarthPosition(V,Phi)

Tfg = coordTransfMatrix(Phi(1),1)*coordTransfMatrix(Phi(2),2)*coordTransfMatrix(Phi(3),3); % Transformation Matrix goedetic --> body reference Frame
Tgf = Tfg';
V_e = Tgf*V;
V_e(3) =  V_e(3);

== matlab function SixDOFSim/6 DOF Linear/Visualisation Non Linear Model Plain 1/MATLAB Function ==
  data: V input; vA output; alpha output; beta output
function [vA,alpha,beta] = getAerodynamical(V)
u = V(1);
v = V(2);
w = V(3);
vA = sqrt(u^2+v^2+w^2);
alpha = atan2(w,u);
beta = asin(v/vA);

== matlab function SixDOFSim/calc_dpsi ==
  data: X input; dpsi output
function dpsi = fcn(X)
q1 = X(5);
r1 = X(6);
phi1 = X(7);
theta1 = X(8);
dpsi1 = (r1*cos(phi1))/cos(theta1) + (q1*sin(phi1))/cos(theta1);

q2 = X(14);
r2 = X(15);
phi2 = X(16);
theta2 = X(17);
dpsi2 = (r2*cos(phi2))/cos(theta2) + (q2*sin(phi2))/cos(theta2);

dpsi = [dpsi1 dpsi2];
end

== matlab function SixDOFSim/6 DOF Non Linear Model Equations/MATLAB Function ==
  data: X input; dX output; U input; psi input; plane_selector input
function dX  = nonlinear_equations_simulink(X,U,psi,plane_selector)
%--------------States------------%
u = X(1);
v = X(2);
w = X(3);
p = X(4);
q = X(5);
r = X(6);
phi = X(7);
theta = X(8);
h = X(9);

%--------------Control------------%
eta = U(1);
sigmaf = U(2);
xi = U(3);
zita = U(4);

%--------------Constants------------%
%% Initialize
g = 9.81; %Gravity [m/s^2]
m = 120000; %Mass [kg]

%Refuel
m_fuel = 28000; %Mass of the fuel
time_refuel = 20; % Time to refuel in sec
start_time_refuel = 10; 
refuel = 0; %Without refuel = 1, with refuel = 0

% Modelling the atmosphere 
rho_const = 1.225; %Airdensity (simplification)
omega_e = 7.29211510*10^(-5); %Rotation Speed of earth [rad/s]
%omega_e = 0;
he = 6356752; %Earth radius [m]
Omega_e_tilde = vecToMat([0;0;omega_e]);

% Inertia and Paramethers of the plane
S = 260; % Flugfläche (wing platform area)
St = 64; %Aerea of the Tail [m^2] 
lt = 24.8; %Length to tail [m] (estimation)
l = 6.6; % generalized length [m]

%Moments of Inertia of Boeing 757-200 [kg(m^2]
% Ix = 10710000; % 
% Ixz = 0; 
% Iy = 14883800; 
% Iz = 25283271; 
% I = [Ix 0 Ixz;0 Iy 0;Ixz 0 Iz]; %Trägheitstensor
I = m*[40.07 0 2.09;0 64 0;2.09 0 99.92];
I_inv = inv(I);

b = 44.8; %Span [m] 
c = 6.6; % Wing Chord [m]

%Aerodynamical Positions
% P_centerGravity = [0.23*c;0;0];
% P_aerodynCenter = [0.12*c;0;0];
P_centerGravity = [0;0;0];
P_aerodynCenter = P_centerGravity;

%Motor and Thrust
%P_thrust = [0.23*c;0;0.1*c+1.9]; %Position of the motor [m] 
P_thrust = [0;0;1.9]; %Position of the motor [m] 
% P_thrust = P_centerGravity;
i_f = 0 ; %Direction of Thrus [rad];
F_max = m*g; %Warning - This is obviusly not the max thrust produced by the turbines. The max Turbine Force is considered on the maximum value of sigmaf

globalParameters.g = g;
globalParameters.m = m;
globalParameters.Omega_e_tilde = Omega_e_tilde;
globalParameters.rho_const = rho_const;
globalParameters.I = I;
globalParameters.I_inv = I_inv;
globalParameters.S = S;
globalParameters.St = St;
globalParameters.lt = lt;
globalParameters.b = b;
globalParameters.c = c;
globalParameters.l = l;
globalParameters.P_thrust =P_thrust;
globalParameters.P_centerGravity = P_centerGravity;
globalParameters.P_aerodynCenter = P_aerodynCenter;
globalParameters.i_f =i_f;
globalParameters.Fmax = F_max;
globalParameters.m_fuel = m_fuel;
globalParameters.time_refuel = time_refuel;
globalParameters.start_time_refuel = start_time_refuel;
globalParameters.refuel = refuel;

%%
T   = 288.15 - 0.0065*h;                    % Temperatur bei H
ps  = 101325*(T/288.15)^(g/1.86584);        % Statischer Luftdruck
rho = ps/(287.053*T);
if plane_selector == 1
    I = globalParameters.I ;
    S = globalParameters.S ;
    St = globalParameters.St ;
    lt = globalParameters.lt ;
    b = globalParameters.b ;
    c = globalParameters.c ;
    P_thrust = globalParameters.P_thrust ;
    P_centerGravity = globalParameters.P_centerGravity ;
    P_aerodynCenter = globalParameters.P_aerodynCenter ;
    i_f = globalParameters.i_f ;
    F_max = globalParameters.Fmax;
elseif plane_selector == 2
    I = globalParameters.I ;
    S = globalParameters.S ;
    St = globalParameters.St ;
    lt = globalParameters.lt ;
    b = globalParameters.b ;
    c = globalParameters.c ;
    P_thrust = globalParameters.P_thrust ;
    P_centerGravity = globalParameters.P_centerGravity ;
    P_aerodynCenter = globalParameters.P_aerodynCenter ;
    i_f = globalParameters.i_f ;
    F_max = globalParameters.Fmax;
end
    
% Airdynamical Coefficients
%CA0 = 1.104;
grad_alpha = 5.5;
alpha_L0 = -11.5*pi/180;
gradient_alpha_epsolon = 0.25;
gradient_CQ_Cbeta = -1.6;
gradientCQ_Czita = 0.24;
CW0 = 0.13;
kappa = 0.07;

% %--------------Variables------------%
% u = sqrt(vA^2*(1-sin(beta)^2)/(1+tan(alpha)^2));
% v = sin(beta)*vA;
% w = u*tan(alpha);
V = [u;v;w];
vA = sqrt(u^2+v^2+w^2);
alpha = atan(w/u);
beta = asin(v/vA);
gamma = theta - alpha;
dh = vA*sin(gamma);

q_d = 0.5*rho*vA^2; %Dynamic Preassure
Omega = [p;q;r];


%--------------Aerodynamical Coefficients------------%
%Forces Coefficients
CA_F = grad_alpha*(alpha - alpha_L0);
epsolon = gradient_alpha_epsolon*(alpha - alpha_L0); %Downwash [rad]
alpha_t = alpha - epsolon + eta +1.3*q*lt/vA; %Angle of Attack of the Tail [rad]
CA_H = 3.1*(St/S)*alpha_t; %Lift Coefficient of the Control Aereas (Elevator-Tail)
CA = CA_F + CA_H; %Total Lift Coefficient

CW = CW0 + kappa*(CA_F - 0.45)^2; %Drag Coefficient

CQ = gradient_CQ_Cbeta*beta + gradientCQ_Czita*zita; % Sideforce coefficient

%Moments Coefficients
N = [-1.4*beta;-0.59-3.1*(St*lt/(l*S))*(alpha-epsolon);(1-alpha*(180/(15*pi)))*beta]; %Static Moments Effects
Jakobi_CM_X = (l/vA)*[-11,    0,           5;
                      0,-4.03*St*lt^2/(S*l^2),0;
                      1.7,          0   , -11.5];
Jakobi_CM_U = [-0.6, 0, 0.22;
               0,    -3.1*St*lt/(S*l),0;
               0, 0, -0.63];      % Dependence of Control Variables
           
C_torque = N + Jakobi_CM_X*Omega + Jakobi_CM_U*[xi;eta;zita];
CL = C_torque(1);
CM = C_torque(2);
CN = C_torque(3);

%-------------- Forces and Moments ------------%
%Aerodynamics
A = q_d*S*CA; %Lift Force [N]
W = q_d*S*CW; %Air Resistance [N]
Q = q_d*S*CQ; %Transverse Force [N]

% EVTL VORZEICHEN VON BETA ÄNDERN
Tfa = coordTransfMatrix(alpha,2)*coordTransfMatrix(-beta,3); %Transformation Matrix Aerodynamics -> Körperfest

RA_a =[-W;Q;-A]; %Aerodynamical Force in Aerdodynamical Reference Frame
RA = Tfa*RA_a; %Aerodynamical Force in Body Reference Frame
QA_aerodynCenter = q_d*S*[b*CL*0.5;c*CM;b*CN*0.5]; %Torque on the aerodynamical Center
QA = QA_aerodynCenter + vecToMat(P_centerGravity- P_aerodynCenter)*RA; %Aerodynamical Force in Body Reference Frame


%Thrust
F_res = F_max*sigmaf; %Thrust Force Absolute Value
Rf = F_res*[cos(i_f);0;sin(i_f)]; %Thrust Force 
Qf = vecToMat(P_thrust - P_centerGravity)*Rf; %Thrust Moment

Q_total = Qf + QA; %Sum of external Moments in Body reference Frame [Nm]
R_total = RA + Rf; %Sum of external Forces in Body reference Frame [N]

%-------------- Equations of Motion ------------%
%Dynamic
Tfg =  coordTransfMatrix(phi,1)*coordTransfMatrix(theta,2)*coordTransfMatrix(psi,3); % Transformation Matrix goedetic --> body reference Frame
Tgf = Tfg.';%Transformation to North East Down
Omega_tilde = vecToMat(Omega);
dOmega = I_inv*(Q_total - Omega_tilde*I*Omega); %Derivative of Rotation Rate (body Reference Frame)

% ACHTUNG: Omega_e_tilde wurde in DGL für dV entfernt, da flache ERde
dV = R_total/m + Tfg*[0;0;g] - (Omega_tilde)*V; %Derivatitive of the Speed (body Reference Frame)
% dvA = (u*dV(1) + v*dV(2) + w*dV(3))/sqrt(u^2 + v^2 + w^2); %Derivative of the Approach Speed
% dalpha = (dV(3)*u - dV(1)*w)/(u^2 + u*w); %Derivative of Angle of Attack
% dbeta = (dV(2)*vA - dvA*V(2))/(vA*sqrt(vA^2 - V(2)^2)); %Derivative of Sideslip Angle

%Kinematics
dP_e = Tgf*V; % gilt nur für z-Komponente

% ACHTUNG: dh anders als im Buch ... Teg fehlt, sollte für dh keinen
% Unterschied machen
% dh = - dP_e(3); %Derivative of z-position (earth Reference Frame)

J = 1/cos(theta)*[cos(theta) sin(phi)*sin(theta) cos(phi)*sin(theta) ;0 cos(phi)*cos(theta) -sin(phi)*cos(theta);0 sin(phi) cos(phi)]; %Rotation rate matrix
dPhi = J*Omega; %Derivative of Euler Angles
dX = double([dV;dOmega;dPhi(1);dPhi(2);dh]);
end
